simulink model "Simulacion_Temporal_LTI"  (R2023b)
settings: Solver=VariableStepAuto  StartTime=0.0  StopTime=1.9  FixedStep=1e-5  MaxStep=1e-5  RelTol=1e-3
values from neighbouring files (symbols this model uses):
  L_q = 5.8e-3    (= 0.0058)    [diagrama_polos_y_ceros_LTI.m]    (also in main.m = 5.8; parametros.m; variacion_de_parametros.m)
  P_p = 3    [Simulacion_Temporal_corrientesytensiones.m]    (also in diagrama_polos_y_ceros_LTI.m; main.m; parametros.m; variacion_de_parametros.m)
libraries: SignalEditorBlockLib x2
settings Model: Creator=Julya  LastModifiedBy=Julya
settings ModelReferenceCC: ModelReferenceMinAlgLoopOccurrences=on

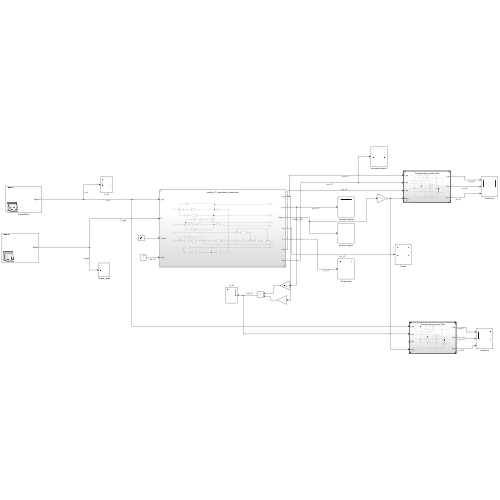
[thumbnail: Simulink's stored preview of the top-level diagram]
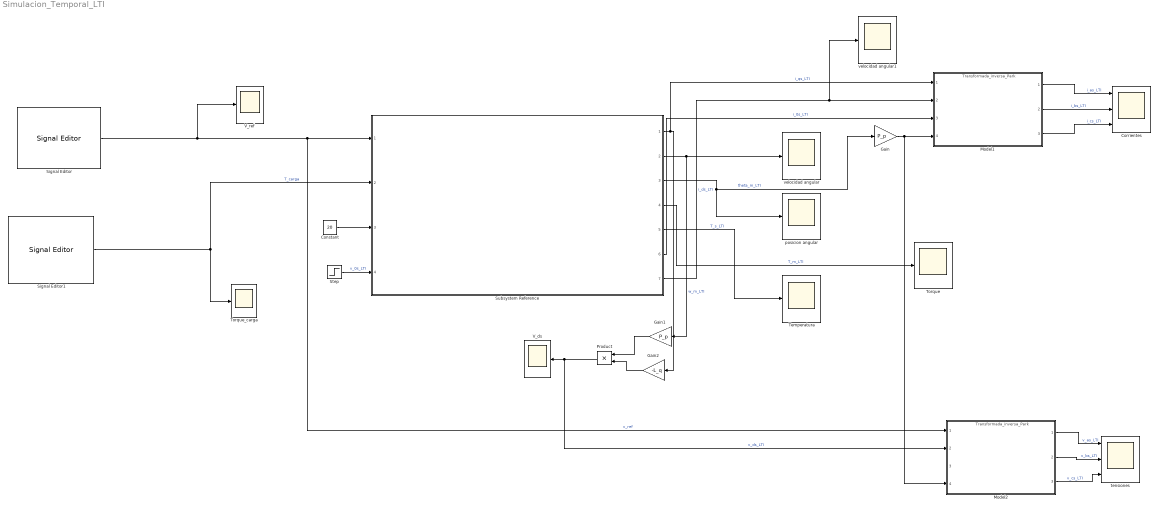
== system Simulacion_Temporal_LTI ==
  Constant : Constant  Value=20
  Corrientes : Scope  NumInputPorts=3
  Gain : Gain  Gain=P_p
  Gain1 : Gain  Gain=P_p
  Gain2 : Gain  Gain=-L_q
  Model1 : ModelReference  ModelNameDialog=Transformada_inversa_Park.slx  SimulationMode=Normal  ModelReferenceVersion=1.6
  Model2 : ModelReference  ModelNameDialog=Transformada_inversa_Park.slx  SimulationMode=Normal  ModelReferenceVersion=1.6
  Product : Product
  Signal Editor : SignalEditorBlockLib/Signal Editor  FileName=V_qs_ref.mat  ActiveScenario=Scenario  ActiveSignal=Signal 1  IsBus=off  OutputBusObjectStr=Bus: BusObject  SampleTime=0  Interpolate=off  ZeroCross=off  OutputAfterFinalValue=Setting to zero  Unit=inherit  PreserveSignalName=on  ApplySigPropsToAllScenarios=on  ApplySigPropsToAllSignals=off
  Signal Editor1 : SignalEditorBlockLib/Signal Editor  FileName=Pulso_Torque_Carga.mat  ActiveScenario=Scenario  ActiveSignal=Signal  IsBus=off  OutputBusObjectStr=Bus: BusObject  SampleTime=0  Interpolate=off  ZeroCross=off  OutputAfterFinalValue=Setting to zero  Unit=inherit  PreserveSignalName=on  ApplySigPropsToAllScenarios=on  ApplySigPropsToAllSignals=off
  Step : Step  Time=0  After=0  SampleTime=0
  Subsystem Reference : Subsystem  ReferencedSubsystem=modelo_LTI_equivalente_aumentado
  Temperatura : Scope
  Torque : Scope
  Torque_carga : Scope
  V_ds : Scope
  V_ref : Scope
  posicion angular : Scope
  tensiones : Scope  NumInputPorts=3
  velocidad angular : Scope
  velocidad angular1 : Scope
  wires:
  Signal Editor/1 -> V_ref/1, Model2/1, Subsystem Reference/1  "v_ref"
  Subsystem Reference/1 -> Gain2/1, Model1/1  "i_qs_LTI"
  Subsystem Reference/2 -> Gain1/1, velocidad angular/1  "w_m_LTI"
  Subsystem Reference/3 -> Gain/1, posicion angular/1  "theta_m_LTI"
  Subsystem Reference/5 -> Temperatura/1  "T_s_LTI"
  Signal Editor1/1 -> Torque_carga/1, Subsystem Reference/2  "T_carga"
  Constant/1 -> Subsystem Reference/3
  Subsystem Reference/4 -> Torque/1  "T_m_LTI"
  Subsystem Reference/6 -> Model1/3  "i_0s_LTI"
  Subsystem Reference/7 -> velocidad angular1/1, Model1/2  "i_ds_LTI"
  Gain/1 -> Model2/4, Model1/4
  Model1/1 -> Corrientes/1  "i_as_LTI"
  Model1/2 -> Corrientes/2  "i_bs_LTI"
  Model1/3 -> Corrientes/3  "i_cs_LTI"
  Gain1/1 -> Product/1
  Gain2/1 -> Product/2
  Product/1 -> Model2/2, V_ds/1  "v_ds_LTI"
  Model2/1 -> tensiones/1  "v_as_LTI"
  Model2/2 -> tensiones/2  "v_bs_LTI"
  Model2/3 -> tensiones/3  "v_cs_LTI"
  Step/1 -> Subsystem Reference/4  "v_0s_LTI"
